simulink model "BPSK"  (R2015a)
settings: Solver=ode45  StartTime=0.0  StopTime=10  RelTol=1e-3
libraries: commdigbbndpm3 x2, commrandsrc2 x2, commchan3 x1, commsink2 x1
settings Model: Creator=Yasmeen  LastModifiedBy=Yasmeen

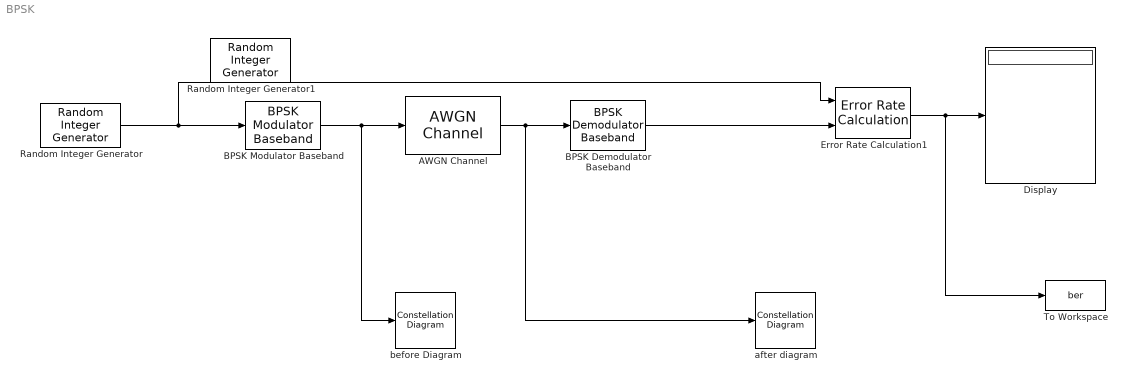
== system BPSK ==
  AWGN Channel : commchan3/AWGN Channel  InputProcessing=Columns as channels (frame based)  seed=67  noiseMode="Signal to noise ratio  (Eb/No)"  EbNodB=EbNo  EsNodB=10  SNRdB=10  bitsPerSym=1  Ps=1  Tsym=1  variance=1
  BPSK Demodulator Baseband : commdigbbndpm3/BPSK Demodulator Baseband  Ph=0  DecType=Hard decision  VarSource=Dialog  Variance=1  outDtype=Inherit via internal rule  derotateFactorWordLen=16
  BPSK Modulator Baseband : commdigbbndpm3/BPSK Modulator Baseband  Ph=0  outDtype=double  outWordLen=16  outUDDataType=sfix(16)  outFracLenMode=Best precision  outFracLen=15
  Display : Display
  Error Rate Calculation1 : commsink2/Error Rate Calculation  N=0  st_delay=0  cp_mode=Entire frame  subframe=[]  PMode=Port  WsName=ErrorVec  RsMode2=off  stop=off  numErr=100  maxBits=1e4
  Random Integer Generator : commrandsrc2/Random Integer Generator  mul=2  seed=37  Ts=1  frameBased=on  sampPerFrame=100  orient=off  outDataType=double
  To Workspace : ToWorkspace  VariableName=ber  SampleTime=-1
      settings: MaxDataPoints=2
  "after diagram " : ConstellationDiagram
  before Diagram : ConstellationDiagram
  Random Integer Generator1 : commrandsrc2/Random Integer Generator  IOType=siggen  mul=8  seed=37  Ts=1  frameBased=off  sampPerFrame=1  orient=off  outDataType=double
  wires:
  Random Integer Generator/1 -> Error Rate Calculation1/1, BPSK Modulator Baseband/1
  BPSK Modulator Baseband/1 -> before Diagram/1, AWGN Channel/1
  AWGN Channel/1 -> "after diagram "/1, BPSK Demodulator Baseband/1
  BPSK Demodulator Baseband/1 -> Error Rate Calculation1/2
  Error Rate Calculation1/1 -> To Workspace/1, Display/1
